simulink model "model"  (R2021b)
settings: Solver=VariableStepAuto  StartTime=0.0  StopTime=10.0  RelTol=1e-3
undefined symbols (not defined in the file or in its folder): b, J, Kb, Kt, L, R
libraries: simulink x1
settings Model: Creator=richa  LastModifiedBy=richa

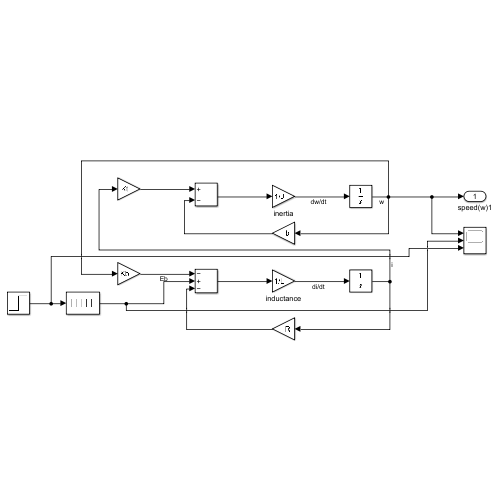
[thumbnail: Simulink's stored preview of the top-level diagram]
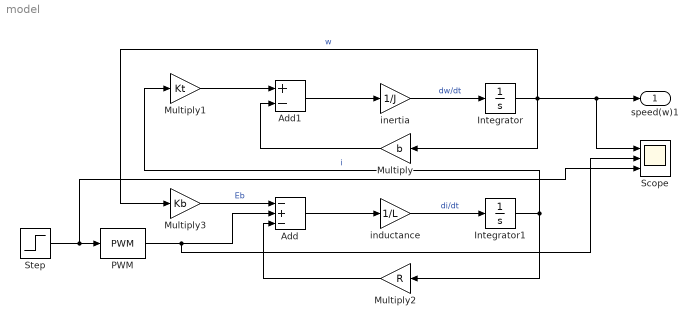
== system model ==
  Add : Sum  Inputs=-+-
  Add1 : Sum  Inputs=+-
  Integrator : Integrator
  Integrator1 : Integrator
  Multiply : Gain  Gain=b
  Multiply1 : Gain  Gain=Kt
  Multiply2 : Gain  Gain=R
  Multiply3 : Gain  Gain=Kb
  PWM : simulink/Discontinuities/PWM  DisableCoverage=on  Period=3  DisallowZeroDutyCycle=off  RunAtFixedTimeIntervals=off  SampleTime=0.1
  Scope : Scope  NumInputPorts=3
  Step : Step  After=0.1  SampleTime=0
  inductance : Gain  Gain=1/L
  inertia : Gain  Gain=1/J
  speed(w)1 : Outport
  wires:
  inertia/1 -> Integrator/1  "dw/dt"
  Step/1 -> PWM/1, Scope/3
  Add/1 -> inductance/1
  inductance/1 -> Integrator1/1  "di/dt"
  Add1/1 -> inertia/1
  Integrator1/1 -> Multiply1/1, Multiply2/1  "i"
  Multiply1/1 -> Add1/1
  Multiply3/1 -> Add/1  "Eb"
  Integrator/1 -> Scope/1, speed(w)1/1, Multiply/1, Multiply3/1  "w"
  Multiply/1 -> Add1/2
  Multiply2/1 -> Add/3
  PWM/1 -> Scope/2, Add/2
